simulink model "signal2Arduino"  (R2017a)
settings: Solver=ode3  StartTime=0.0  StopTime=T_end  FixedStep=Ts_sim  RelTol=1e-3  EnableMultiTasking=on
undefined symbols (not defined in the file or in its folder): A_butter_acc, A_butter_cal, A_butter_low, AD622, B_butter_acc, B_butter_cal, B_butter_low, b_stop, delta_EMG_RT, delta_theta1, EMG2vel_gain, g, Humusoft, input_type, k_stop, Ki_vel, Kp_vel, L_com, m1, m3, m_arm, min_EMG_RT, National_Instruments, PCI, phase_experiment, q1, q3, tau_max_cont, thetaL1_max, thetaL1_min, thetaR1_max, thetaR1_min, Ts_acc, Ts_sim, X, Y, Z
libraries: sm_lib x56, nesl_utility x23, sldrtlib x18, instrumentlib x2, simulink x1
(part 1 of 2)
settings Model: ExtModeTrigDuration=2  Creator=Fred Parietti  LastModifiedBy=jacob
settings DataIOCC: LimitDataPoints=on  SaveFormat=Array
settings OptimizationCC: LifeSpan=1
settings DebuggingCC: UnderspecifiedInitializationDetection=Classic  MergeDetectMultiDrivingBlocksExec=none  SFUnexpectedBacktrackingDiag=warning  SFNoUnconditionalDefaultTransitionDiag=warning  SFExecutionAtInitializationDiag=none
settings HardwareCC: ProdBitPerInt=16  ProdBitPerPointer=8  ProdBitPerSizeT=16  ProdBitPerPtrDiffT=16  ProdLargestAtomicFloat=None  ProdWordSize=8  ProdHWDeviceType=Atmel->AVR
settings ModelReferenceCC: PropagateSignalLabelsOutOfModel=off
settings SFSimCC: MATLABDynamicMemAlloc=off
settings RTWCC: SystemTargetFile=realtime.tlc  GenerateMakefile=off  TemplateMakefile=realtime.tmf  Description=Run on Target Hardware  RTWVerbose=off
settings STFCustomTargetCC: TargetLibSuffix=.a  GenerateSampleERTMain=on  ERTCustomFileBanners=on  SupportNonInlinedSFcns=off  RemoveResetFunc=on  SupportVariableSizeSignals=on  MATLABClassNameForMDSCustomization=Simulink.SoftwareTarget.ERTCustomization  GRTInterface=off  SystemTargetFile=realtime.tlc
settings ERTTargetCC: MultiwordLength=2048  GenerateSampleERTMain=on  ParMdlRefBuildCompliant=off  CompOptLevelCompliant=off  ConcurrentExecutionCompliant=off  CombineOutputUpdateFcns=off  ERTFirstTimeCompliant=off  SupportContinuousTime=on  SupportVariableSizeSignals=on  ModelStepFunctionPrototypeControlCompliant=off  CPPClassGenCompliant=off  UseToolchainInfoCompliant=off  ExtModeTransport=3  ExtModeMexFile=ext_serial_win32_comm_rtt  ExtModeMexArgs=0 1 9600  ERTSrcFileBannerTemplate=realtime_code_template.cgt  ERTHdrFileBannerTemplate=realtime_code_template.cgt  ERTDataSrcFileTemplate=realtime_code_template.cgt  ERTDataHdrFileTemplate=realtime_code_template.cgt  ERTCustomFileTemplate=realtime_file_process.tlc  ConvertIfToSwitch=off  SuppressUnreachableDefaultCases=off
settings ConfigComp: CovMetricSettings=dw  CovHtmlReporting=on  CovSaveCumulativeToWorkspaceVar=on  CovSaveSingleToWorkspaceVar=on  CovExternalEMLEnable=off
settings ConfigurationSet: Description=SimMechanics 2G
settings ExplorerConfigSet: InternalSimMechanicsExplorerSettings="<ExplorerConfiguration><canonicalview>planar_xy</canonicalview><AnimationSetting><BasePlaybackSpeed>1.0</BasePlaybackSpeed><PlaybackSpeedFactor>1.0</PlaybackSpeedFactor></AnimationSetting><TilePanel><TileInfo><Tiles Columns=\"1\" Count=\"1\" Rows=\"1\"><Column Left=\"2\" Weight=\"1\"/><Column Left=\"1036\"/><Row Top=\"2\" Weight=\"1\"/><Row Top=\"856\"/><Tile Height=\"1\" Width=\"1\" X=\"0\" Y=\"0\"/></Tiles></TileInfo><SceneInfo><SceneViewer><BGColor><R>1</R><G>1</G><B>1</B></BGColor><Camera><Position><X>1.1720425313593452</X><Y>1.5909414689803159</Y><Z>2.2841318134829445</Z></Position><Center><X>-0.16046430282016899</X><Y>0.25843463480080253</Y><Z>0.95162497930343193</Z></Center><Up><X>-0.40824829046386307</X><Y>0.81649658092772615</Y><Z>-0.40824829046386307</Z></Up><Left>-1.5455518852644918</Left><Right>1.5455518852644918</Right><Bottom>-1.165175562863084</Bottom><Top>1.165175562863084</Top></Camera></SceneViewer></SceneInfo></TilePanel></ExplorerConfiguration>"

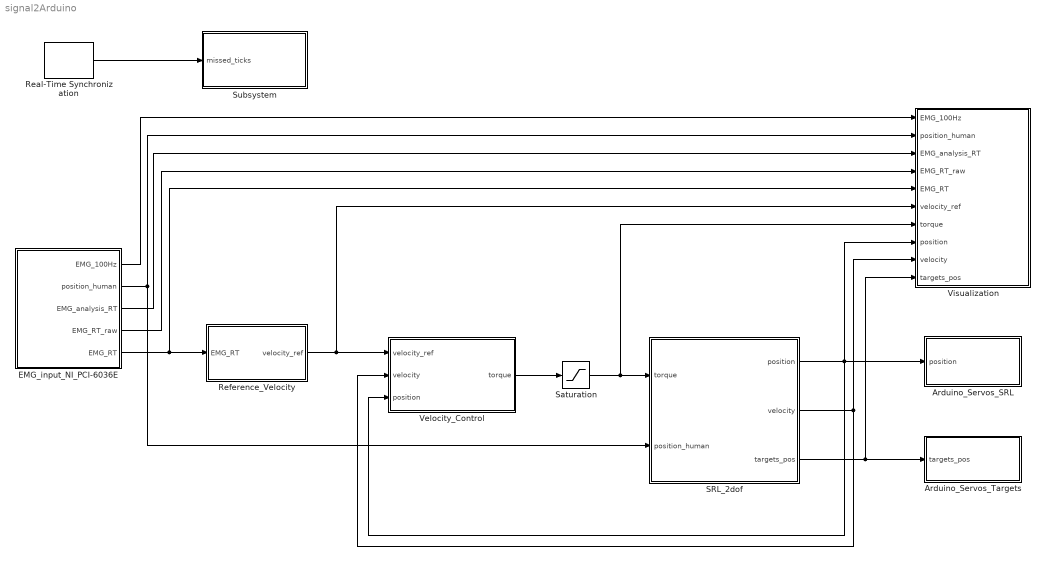
== system signal2Arduino ==
  Arduino_Servos_SRL : Subsystem
  Arduino_Servos_Targets : Subsystem
  EMG_input_NI_PCI-6036E : Subsystem
  Real-Time Synchronization : sldrtlib/Real-Time Synchronization  SampleTime=Ts_sim  MaxMissedTicks=10000  ShowMissedTicks=on  YieldWhenWaiting=off
  Reference_Velocity : Subsystem
  SRL_2dof : Subsystem
  Saturation : Saturate  UpperLimit=tau_max_cont  LowerLimit=-tau_max_cont
  Subsystem : Subsystem
  Velocity_Control : Subsystem
  Visualization : Subsystem
  wires:
  SRL_2dof/1(position) -> Velocity_Control/3(position), Arduino_Servos_SRL/1(position), Visualization/8(position)
  Saturation/1 -> Visualization/7(torque), SRL_2dof/1(torque)
  SRL_2dof/2(velocity) -> Velocity_Control/2(velocity), Visualization/9(velocity)
  Reference_Velocity/1(velocity_ref) -> Velocity_Control/1(velocity_ref), Visualization/6(velocity_ref)
  Velocity_Control/1(torque) -> Saturation/1
  EMG_input_NI_PCI-6036E/5(EMG_RT) -> Visualization/5(EMG_RT), Reference_Velocity/1(EMG_RT)
  Real-Time Synchronization/1 -> Subsystem/1(missed_ticks)
  SRL_2dof/3(targets_pos) -> Visualization/10(targets_pos), Arduino_Servos_Targets/1(targets_pos)
  EMG_input_NI_PCI-6036E/3(EMG_analysis_RT) -> Visualization/3(EMG_analysis_RT)
  EMG_input_NI_PCI-6036E/2(position_human) -> Visualization/2(position_human), SRL_2dof/2(position_human)
  EMG_input_NI_PCI-6036E/4(EMG_RT_raw) -> Visualization/4(EMG_RT_raw)
  EMG_input_NI_PCI-6036E/1(EMG_100Hz) -> Visualization/1(EMG_100Hz)

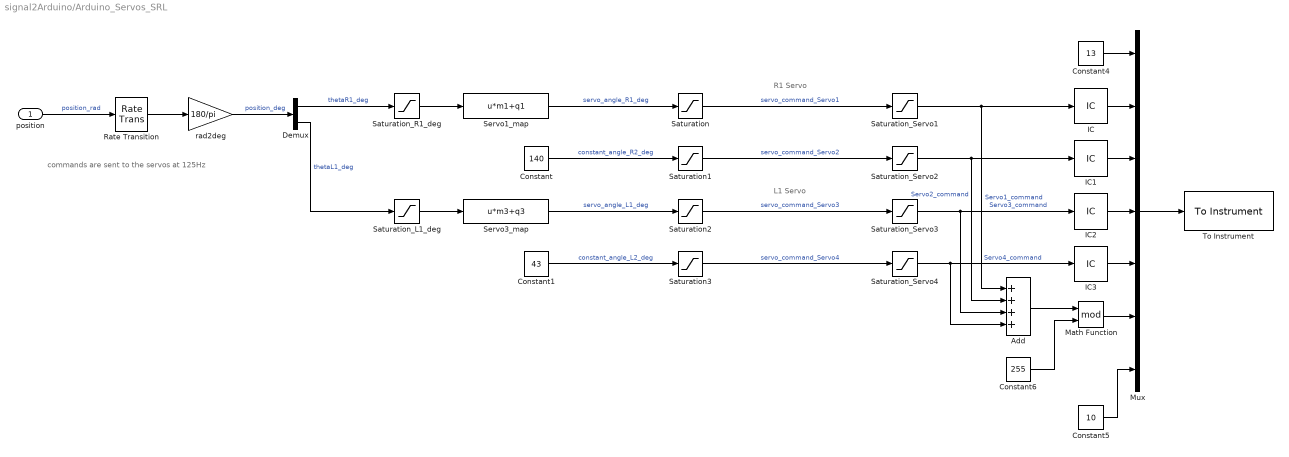
== system signal2Arduino/Arduino_Servos_SRL ==
  note: R1 Servo
  note: L1 Servo
  note: commands are sent to the servos at 125Hz
  position : Inport
  Add : Sum  Inputs=++++
  Constant : Constant  Value=140
  Constant1 : Constant  Value=43
  Constant4 : Constant  Value=13
  Constant5 : Constant  Value=10
  Constant6 : Constant  Value=255
  Demux : Demux  Outputs=2
  IC{,1..3} (4 alike) : InitialCondition  Value=90
  Math Function : Math  Operator=mod  SaturateOnIntegerOverflow=on
  Mux : Mux  Inputs=7
  Rate Transition : RateTransition  Deterministic=off  OutPortSampleTime=0.008
  Saturation : Saturate  UpperLimit=150  LowerLimit=23
  Saturation1 : Saturate  UpperLimit=140  LowerLimit=90
  Saturation2 : Saturate  UpperLimit=158  LowerLimit=30
  Saturation3 : Saturate  UpperLimit=93  LowerLimit=43
  Saturation_L1_deg : Saturate  UpperLimit=thetaL1_max/pi*180  LowerLimit=thetaL1_min/pi*180
  Saturation_R1_deg : Saturate  UpperLimit=thetaR1_max/pi*180  LowerLimit=thetaR1_min/pi*180
  Saturation_Servo{1..4} (4 alike) : Saturate  UpperLimit=180  LowerLimit=0
  Servo1_map : Fcn  Expr=u*m1+q1
  Servo3_map : Fcn  Expr=u*m3+q3
  To Instrument : instrumentlib/To Instrument  sampleTime=0.008  isWorkspaceObject=on  timeout=10  inputBufferSize=8192  protocol=Serial  serialPort=COM1  baudRate=9600  gpibVendor=Agilent Technologies  boardIndex=0  primaryAddress=1  secondaryAddress=0  visaVendor=Agilent  visaSerialPort=0  chassisIndex=0  logicalAddress=0  tcpRemoteHost='127.0.0.1'  tcpRemotePort=4500  udpRemoteHost='127.0.0.1'  udpRemotePort=9090  visaTCPBoardIndex=0  visaTCPRemoteHost='127.0.0.1'  usbBoardIndex=0  usbManufID=0  usbModelCode=0  usbSerialNumber=0  wsVariableName=s_SRL  initAction=None  initCommand='DATA:SOURCE CH1'  initFunction=get  command=''  sendFormat=Binary  asciiFormatting='%d'  precision=8-bit unsigned integer  byteOrder=Little endian
      settings: SourceProductName=Instrument Control Toolbox  SourceProductBaseCode=IC
  rad2deg : Gain  Gain=180/pi
  wires:
  position/1 -> Rate Transition/1  "position_rad"
  rad2deg/1 -> Demux/1  "position_deg"
  Demux/1 -> Saturation_R1_deg/1  "thetaR1_deg"
  Servo1_map/1 -> Saturation/1  "servo_angle_R1_deg"
  Demux/2 -> Saturation_L1_deg/1  "thetaL1_deg"
  Servo3_map/1 -> Saturation2/1  "servo_angle_L1_deg"
  Rate Transition/1 -> rad2deg/1
  Saturation/1 -> Saturation_Servo1/1  "servo_command_Servo1"
  Saturation1/1 -> Saturation_Servo2/1  "servo_command_Servo2"
  Saturation2/1 -> Saturation_Servo3/1  "servo_command_Servo3"
  Saturation3/1 -> Saturation_Servo4/1  "servo_command_Servo4"
  Constant/1 -> Saturation1/1  "constant_angle_R2_deg"
  Constant1/1 -> Saturation3/1  "constant_angle_L2_deg"
  Saturation_R1_deg/1 -> Servo1_map/1
  Saturation_L1_deg/1 -> Servo3_map/1
  Saturation_Servo4/1 -> IC3/1, Add/4  "Servo4_command"
  Saturation_Servo3/1 -> IC2/1, Add/3  "Servo3_command"
  Saturation_Servo2/1 -> IC1/1, Add/2  "Servo2_command"
  Saturation_Servo1/1 -> Add/1, IC/1  "Servo1_command"
  Math Function/1 -> Mux/6
  Constant4/1 -> Mux/1
  Constant6/1 -> Math Function/2
  Add/1 -> Math Function/1
  Constant5/1 -> Mux/7
  Mux/1 -> To Instrument/1
  IC/1 -> Mux/2
  IC1/1 -> Mux/3
  IC2/1 -> Mux/4
  IC3/1 -> Mux/5

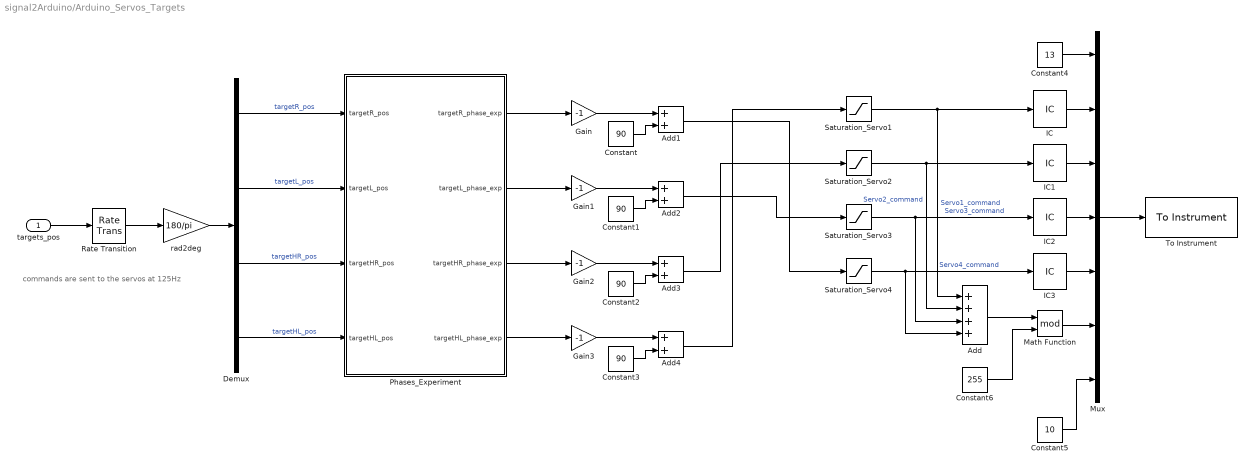
== system signal2Arduino/Arduino_Servos_Targets ==
  note: commands are sent to the servos at 125Hz
  targets_pos : Inport
  Add : Sum  Inputs=++++
  Add{1..4} (4 alike) : Sum
  Constant{,1..3} (4 alike) : Constant  Value=90
  Constant4 : Constant  Value=13
  Constant5 : Constant  Value=10
  Constant6 : Constant  Value=255
  Demux : Demux
  Gain{,1..3} (4 alike) : Gain  Gain=-1
  IC{,1..3} (4 alike) : InitialCondition  Value=90
  Math Function : Math  Operator=mod  SaturateOnIntegerOverflow=on
  Mux : Mux  Inputs=7
  Phases_Experiment : Subsystem
  Rate Transition : RateTransition  Deterministic=off  OutPortSampleTime=0.008
  Saturation_Servo{1..4} (4 alike) : Saturate  UpperLimit=180  LowerLimit=0
  To Instrument : instrumentlib/To Instrument  sampleTime=0.008  isWorkspaceObject=on  timeout=10  inputBufferSize=8192  protocol=Serial  serialPort=COM1  baudRate=9600  gpibVendor=Agilent Technologies  boardIndex=0  primaryAddress=1  secondaryAddress=0  visaVendor=Agilent  visaSerialPort=0  chassisIndex=0  logicalAddress=0  tcpRemoteHost='127.0.0.1'  tcpRemotePort=4500  udpRemoteHost='127.0.0.1'  udpRemotePort=9090  visaTCPBoardIndex=0  visaTCPRemoteHost='127.0.0.1'  usbBoardIndex=0  usbManufID=0  usbModelCode=0  usbSerialNumber=0  wsVariableName=s_targets  initAction=None  initCommand='DATA:SOURCE CH1'  initFunction=get  command=''  sendFormat=Binary  asciiFormatting='%d'  precision=8-bit unsigned integer  byteOrder=Little endian
      settings: SourceProductName=Instrument Control Toolbox  SourceProductBaseCode=IC
  rad2deg : Gain  Gain=180/pi
  wires:
  Saturation_Servo4/1 -> IC3/1, Add/4  "Servo4_command"
  Saturation_Servo3/1 -> IC2/1, Add/3  "Servo3_command"
  Saturation_Servo2/1 -> IC1/1, Add/2  "Servo2_command"
  Saturation_Servo1/1 -> Add/1, IC/1  "Servo1_command"
  Math Function/1 -> Mux/6
  Constant4/1 -> Mux/1
  Constant6/1 -> Math Function/2
  Add/1 -> Math Function/1
  Constant5/1 -> Mux/7
  Mux/1 -> To Instrument/1
  targets_pos/1 -> Rate Transition/1
  Demux/1 -> Phases_Experiment/1(targetR_pos)  "targetR_pos"
  Gain/1 -> Add1/1
  rad2deg/1 -> Demux/1
  Constant/1 -> Add1/2
  Gain1/1 -> Add2/1
  Constant1/1 -> Add2/2
  Gain2/1 -> Add3/1
  Constant2/1 -> Add3/2
  Gain3/1 -> Add4/1
  Constant3/1 -> Add4/2
  Demux/3 -> Phases_Experiment/3(targetHR_pos)  "targetHR_pos"
  Demux/2 -> Phases_Experiment/2(targetL_pos)  "targetL_pos"
  Demux/4 -> Phases_Experiment/4(targetHL_pos)  "targetHL_pos"
  Rate Transition/1 -> rad2deg/1
  IC/1 -> Mux/2
  IC1/1 -> Mux/3
  IC2/1 -> Mux/4
  IC3/1 -> Mux/5
  Add1/1 -> Saturation_Servo4/1
  Add2/1 -> Saturation_Servo3/1
  Add3/1 -> Saturation_Servo2/1
  Add4/1 -> Saturation_Servo1/1
  Phases_Experiment/1(targetR_phase_exp) -> Gain/1
  Phases_Experiment/2(targetL_phase_exp) -> Gain1/1
  Phases_Experiment/3(targetHR_phase_exp) -> Gain2/1
  Phases_Experiment/4(targetHL_phase_exp) -> Gain3/1

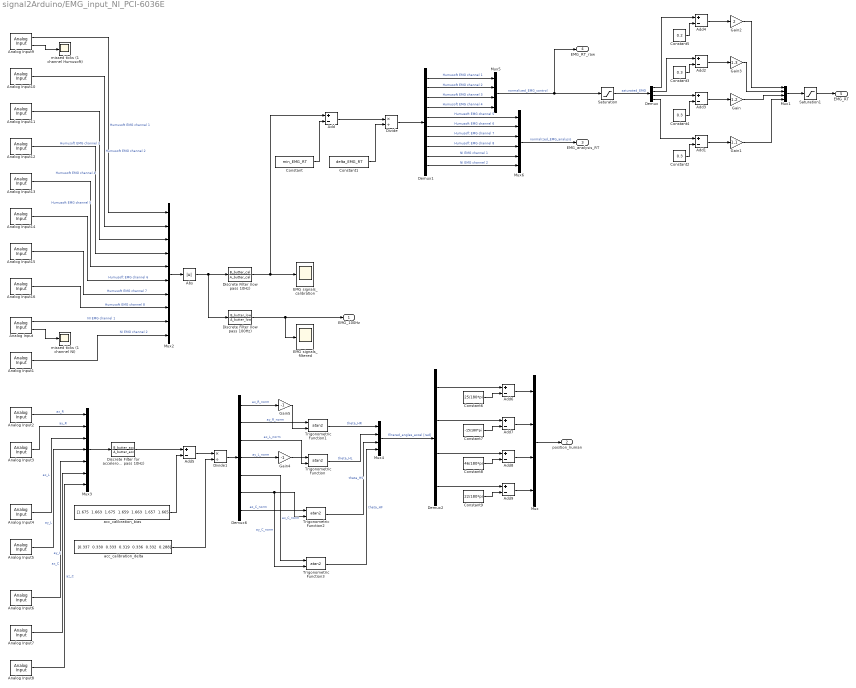
== system signal2Arduino/EMG_input_NI_PCI-6036E ==
  Abs : Abs
  Add{,1..9} (10 alike) : Sum  Inputs=+-
  Analog Input : sldrtlib/Analog Input  SampleTime=Ts_sim  MaxMissedTicks=10000  ShowMissedTicks=on  YieldWhenWaiting=off  DrvName=National_Instruments/PCI-6036E  DrvAddress=4294967295  DrvOptions=[0 0 0 0 0 0]  Channels=1  RangeMode=1  VoltRange=1  DataType=1
      settings: AttributesFormatString=National Instruments\nPCI-6036E [auto]  SourceProductName=Simulink Desktop Real-Time
  Analog Input1 : sldrtlib/Analog Input  SampleTime=Ts_sim  MaxMissedTicks=10000  ShowMissedTicks=off  YieldWhenWaiting=off  DrvName=National_Instruments/PCI-6036E  DrvAddress=4294967295  DrvOptions=[0 0 0 0 0 0]  Channels=2  RangeMode=1  VoltRange=1  DataType=1
      settings: AttributesFormatString=National Instruments\nPCI-6036E [auto]  SourceProductName=Simulink Desktop Real-Time
  Analog Input10 : sldrtlib/Analog Input  SampleTime=Ts_sim  MaxMissedTicks=10000  ShowMissedTicks=off  YieldWhenWaiting=off  DrvName=Humusoft/AD622  DrvAddress=4294967295  DrvOptions=zeros(1,0)  Channels=2  RangeMode=1  VoltRange=1  DataType=1
      settings: AttributesFormatString=Humusoft\nAD622 [auto]  SourceProductName=Simulink Desktop Real-Time
  Analog Input11 : sldrtlib/Analog Input  SampleTime=Ts_sim  MaxMissedTicks=10000  ShowMissedTicks=off  YieldWhenWaiting=off  DrvName=Humusoft/AD622  DrvAddress=4294967295  DrvOptions=zeros(1,0)  Channels=3  RangeMode=1  VoltRange=1  DataType=1
      settings: AttributesFormatString=Humusoft\nAD622 [auto]  SourceProductName=Simulink Desktop Real-Time
  Analog Input12 : sldrtlib/Analog Input  SampleTime=Ts_sim  MaxMissedTicks=10000  ShowMissedTicks=off  YieldWhenWaiting=off  DrvName=Humusoft/AD622  DrvAddress=4294967295  DrvOptions=zeros(1,0)  Channels=4  RangeMode=1  VoltRange=1  DataType=1
      settings: AttributesFormatString=Humusoft\nAD622 [auto]  SourceProductName=Simulink Desktop Real-Time
  Analog Input13 : sldrtlib/Analog Input  SampleTime=Ts_sim  MaxMissedTicks=10000  ShowMissedTicks=off  YieldWhenWaiting=off  DrvName=Humusoft/AD622  DrvAddress=4294967295  DrvOptions=zeros(1,0)  Channels=5  RangeMode=1  VoltRange=1  DataType=1
      settings: AttributesFormatString=Humusoft\nAD622 [auto]  SourceProductName=Simulink Desktop Real-Time
  Analog Input14 : sldrtlib/Analog Input  SampleTime=Ts_sim  MaxMissedTicks=10000  ShowMissedTicks=off  YieldWhenWaiting=off  DrvName=Humusoft/AD622  DrvAddress=4294967295  DrvOptions=zeros(1,0)  Channels=6  RangeMode=1  VoltRange=1  DataType=1
      settings: AttributesFormatString=Humusoft\nAD622 [auto]  SourceProductName=Simulink Desktop Real-Time
  Analog Input15 : sldrtlib/Analog Input  SampleTime=Ts_sim  MaxMissedTicks=10000  ShowMissedTicks=off  YieldWhenWaiting=off  DrvName=Humusoft/AD622  DrvAddress=4294967295  DrvOptions=zeros(1,0)  Channels=7  RangeMode=1  VoltRange=1  DataType=1
      settings: AttributesFormatString=Humusoft\nAD622 [auto]  SourceProductName=Simulink Desktop Real-Time
  Analog Input16 : sldrtlib/Analog Input  SampleTime=Ts_sim  MaxMissedTicks=10000  ShowMissedTicks=off  YieldWhenWaiting=off  DrvName=Humusoft/AD622  DrvAddress=4294967295  DrvOptions=zeros(1,0)  Channels=8  RangeMode=1  VoltRange=1  DataType=1
      settings: AttributesFormatString=Humusoft\nAD622 [auto]  SourceProductName=Simulink Desktop Real-Time
  Analog Input2 : sldrtlib/Analog Input  SampleTime=Ts_acc  MaxMissedTicks=10000  ShowMissedTicks=off  YieldWhenWaiting=off  DrvName=National_Instruments/PCI-6036E  DrvAddress=4294967295  DrvOptions=[0 0 0 0 0 0]  Channels=3  RangeMode=1  VoltRange=1  DataType=1
      settings: AttributesFormatString=National Instruments\nPCI-6036E [auto]  SourceProductName=Simulink Desktop Real-Time
  Analog Input3 : sldrtlib/Analog Input  SampleTime=Ts_acc  MaxMissedTicks=10000  ShowMissedTicks=off  YieldWhenWaiting=off  DrvName=National_Instruments/PCI-6036E  DrvAddress=4294967295  DrvOptions=[0 0 0 0 0 0]  Channels=4  RangeMode=1  VoltRange=1  DataType=1
      settings: AttributesFormatString=National Instruments\nPCI-6036E [auto]  SourceProductName=Simulink Desktop Real-Time
  Analog Input4 : sldrtlib/Analog Input  SampleTime=Ts_acc  MaxMissedTicks=10000  ShowMissedTicks=off  YieldWhenWaiting=off  DrvName=National_Instruments/PCI-6036E  DrvAddress=4294967295  DrvOptions=[0 0 0 0 0 0]  Channels=5  RangeMode=1  VoltRange=1  DataType=1
      settings: AttributesFormatString=National Instruments\nPCI-6036E [auto]  SourceProductName=Simulink Desktop Real-Time
  Analog Input5 : sldrtlib/Analog Input  SampleTime=Ts_acc  MaxMissedTicks=10000  ShowMissedTicks=off  YieldWhenWaiting=off  DrvName=National_Instruments/PCI-6036E  DrvAddress=4294967295  DrvOptions=[0 0 0 0 0 0]  Channels=6  RangeMode=1  VoltRange=1  DataType=1
      settings: AttributesFormatString=National Instruments\nPCI-6036E [auto]  SourceProductName=Simulink Desktop Real-Time
  Analog Input6 : sldrtlib/Analog Input  SampleTime=Ts_acc  MaxMissedTicks=10000  ShowMissedTicks=off  YieldWhenWaiting=off  DrvName=National_Instruments/PCI-6036E  DrvAddress=4294967295  DrvOptions=[0 0 0 0 0 0]  Channels=7  RangeMode=1  VoltRange=1  DataType=1
      settings: AttributesFormatString=National Instruments\nPCI-6036E [auto]  SourceProductName=Simulink Desktop Real-Time
  Analog Input7 : sldrtlib/Analog Input  SampleTime=Ts_acc  MaxMissedTicks=10000  ShowMissedTicks=off  YieldWhenWaiting=off  DrvName=National_Instruments/PCI-6036E  DrvAddress=4294967295  DrvOptions=[0 0 0 0 0 0]  Channels=8  RangeMode=1  VoltRange=1  DataType=1
      settings: AttributesFormatString=National Instruments\nPCI-6036E [auto]  SourceProductName=Simulink Desktop Real-Time
  Analog Input8 : sldrtlib/Analog Input  SampleTime=Ts_acc  MaxMissedTicks=10000  ShowMissedTicks=off  YieldWhenWaiting=off  DrvName=National_Instruments/PCI-6036E  DrvAddress=4294967295  DrvOptions=[0 0 0 0 0 0]  Channels=16  RangeMode=1  VoltRange=1  DataType=1
      settings: AttributesFormatString=National Instruments\nPCI-6036E [auto]  SourceProductName=Simulink Desktop Real-Time
  Analog Input9 : sldrtlib/Analog Input  SampleTime=Ts_sim  MaxMissedTicks=10000  ShowMissedTicks=on  YieldWhenWaiting=off  DrvName=Humusoft/AD622  DrvAddress=4294967295  DrvOptions=zeros(1,0)  Channels=1  RangeMode=1  VoltRange=1  DataType=1
      settings: AttributesFormatString=Humusoft\nAD622 [auto]  SourceProductName=Simulink Desktop Real-Time
  Constant : Constant  Value=min_EMG_RT
  Constant1 : Constant  Value=delta_EMG_RT
  Constant2 : Constant  Value=0.3
  Constant3 : Constant  Value=0.3
  Constant4 : Constant  Value=0.3
  Constant5 : Constant  Value=0.2
  Constant6 : Constant  Value=25/180*pi
  Constant7 : Constant  Value=-15/180*pi
  Constant8 : Constant  Value=46/180*pi
  Constant9 : Constant  Value=22/180*pi
  Demux : Demux
  Demux1 : Demux  Outputs=10
  Demux2 : Demux
  Demux6 : Demux  Outputs=7
  Discrete Filter (low pass 100Hz) : DiscreteFilter  Numerator=B_butter_low  Denominator=A_butter_low
  Discrete Filter (low pass 10Hz) : DiscreteFilter  Numerator=B_butter_cal  Denominator=A_butter_cal
  Discrete Filter for accelerometers (low pass 10Hz) : DiscreteFilter  Numerator=B_butter_acc  Denominator=A_butter_acc
  Divide : Product  Inputs=*/
  Divide1 : Product  Inputs=*/
  EMG signals_calibration : Scope
  EMG signals_filtered : Scope
  Gain : Gain  Gain=1.2
  Gain1 : Gain  Gain=1.1
  Gain2 : Gain  Gain=2
  Gain3 : Gain  Gain=1.3
  Gain4 : Gain  Gain=-1
  Gain5 : Gain  Gain=-1
  Mux{,1,4..5} (4 alike) : Mux
  Mux2 : Mux  Inputs=10
  Mux3 : Mux  Inputs=7
  Mux6 : Mux  Inputs=6
  Saturation : Saturate  UpperLimit=1  LowerLimit=0
  Saturation1 : Saturate  UpperLimit=1  LowerLimit=0
  Trigonometric Function{,1..3} (4 alike) : Trigonometry  Operator=atan2
  acc_calibration_bias : Constant  Value="[1.675  1.663  1.675  1.659  1.663  1.657  1.665]"
  acc_calibration_delta : Constant  Value="[0.337  0.330  0.333  0.319  0.336  0.332  0.288]"
  missed ticks (1 channel Humusoft) : Scope
  missed ticks (1 channel NI) : Scope
  EMG_100Hz : Outport
  position_human : Outport  Port=2
  EMG_analysis_RT : Outport  Port=3
  EMG_RT_raw : Outport  Port=4
  EMG_RT : Outport  Port=5
  wires:
  Constant/1 -> Add/2
  Add/1 -> Divide/1
  Constant1/1 -> Divide/2
  Saturation/1 -> Demux/1  "saturated_EMG"
  Demux/4 -> Add1/1
  Constant2/1 -> Add1/2
  Demux/1 -> Add4/1
  Add1/1 -> Gain1/1
  Mux1/1 -> Saturation1/1
  Demux/2 -> Add2/1
  Constant3/1 -> Add2/2
  Add2/1 -> Gain3/1
  Saturation1/1 -> EMG_RT/1
  Demux/3 -> Add3/1
  Add3/1 -> Gain/1
  Constant4/1 -> Add3/2
  Constant5/1 -> Add4/2
  Add4/1 -> Gain2/1
  Gain/1 -> Mux1/3
  Gain1/1 -> Mux1/4
  Gain2/1 -> Mux1/1
  Gain3/1 -> Mux1/2
  Analog Input/1 -> Mux2/9  "NI EMG channel 1"
  Analog Input/2 -> missed ticks (1 channel NI)/1
  Analog Input1/1 -> Mux2/10  "NI EMG channel 2"
  Discrete Filter (low pass 10Hz)/1 -> Add/1, EMG signals_calibration/1
  Mux3/1 -> Discrete Filter for accelerometers (low pass 10Hz)/1
  Demux6/3 -> Trigonometric Function/2  "ax_L_norm"
  Demux6/4 -> Gain4/1  "ay_L_norm"
  Gain4/1 -> Trigonometric Function/1
  Trigonometric Function/1 -> Mux4/2  "theta_HL"
  Add5/1 -> Divide1/1
  Demux6/1 -> Gain5/1  "ax_R_norm"
  Demux6/2 -> Trigonometric Function1/1  "ay_R_norm"
  Trigonometric Function1/1 -> Mux4/1  "theta_HR"
  Divide1/1 -> Demux6/1
  Gain5/1 -> Trigonometric Function1/2
  Demux6/5 -> Trigonometric Function3/1  "ax_C_norm"
  Demux6/6 -> Trigonometric Function3/2, Trigonometric Function2/2  "ay_C_norm"
  Demux6/7 -> Trigonometric Function2/1  "az_C_norm"
  Trigonometric Function2/1 -> Mux4/3  "theta_HS"
  Trigonometric Function3/1 -> Mux4/4  "theta_HF"
  Analog Input2/1 -> Mux3/1  "ax_R"
  Analog Input3/1 -> Mux3/2  "ay_R"
  Analog Input4/1 -> Mux3/3  "ax_L"
  Analog Input5/1 -> Mux3/4  "ay_L"
  Analog Input6/1 -> Mux3/5  "ax_C"
  Analog Input7/1 -> Mux3/6  "ay_C"
  Analog Input8/1 -> Mux3/7  "az_C"
  Mux2/1 -> Abs/1
  Analog Input9/2 -> missed ticks (1 channel Humusoft)/1
  Analog Input9/1 -> Mux2/1  "Humusoft EMG channel 1"
  Analog Input10/1 -> Mux2/2  "Humusoft EMG channel 2"
  Analog Input11/1 -> Mux2/3  "Humusoft EMG channel 3"
  Analog Input12/1 -> Mux2/4  "Humusoft EMG channel 4"
  Analog Input13/1 -> Mux2/5  "Humusoft EMG channel 5"
  Analog Input16/1 -> Mux2/8  "Humusoft EMG channel 8"
  Analog Input14/1 -> Mux2/6  "Humusoft EMG channel 6"
  Analog Input15/1 -> Mux2/7  "Humusoft EMG channel 7"
  Mux4/1 -> Demux2/1  "filtered_angles_accel [rad]"
  Discrete Filter for accelerometers (low pass 10Hz)/1 -> Add5/1
  Abs/1 -> Discrete Filter (low pass 10Hz)/1, Discrete Filter (low pass 100Hz)/1
  Discrete Filter (low pass 100Hz)/1 -> EMG_100Hz/1, EMG signals_filtered/1
  Demux1/1 -> Mux5/1  "Humusoft EMG channel 1"
  Demux1/2 -> Mux5/2  "Humusoft EMG channel 2"
  Demux1/3 -> Mux5/3  "Humusoft EMG channel 3"
  Demux1/4 -> Mux5/4  "Humusoft EMG channel 4"
  Mux5/1 -> EMG_RT_raw/1, Saturation/1  "normalized_EMG_control"
  Demux1/5 -> Mux6/1  "Humusoft EMG channel 5"
  Demux1/10 -> Mux6/6  "NI EMG channel 2"
  Demux1/6 -> Mux6/2  "Humusoft EMG channel 6"
  Demux1/7 -> Mux6/3  "Humusoft EMG channel 7"
  Demux1/8 -> Mux6/4  "Humusoft EMG channel 8"
  Demux1/9 -> Mux6/5  "NI EMG channel 1"
  Mux6/1 -> EMG_analysis_RT/1  "normalized_EMG_analysis"
  Divide/1 -> Demux1/1
  acc_calibration_bias/1 -> Add5/2
  acc_calibration_delta/1 -> Divide1/2
  Mux/1 -> position_human/1
  Demux2/1 -> Add6/1
  Constant6/1 -> Add6/2
  Demux2/2 -> Add7/1
  Constant7/1 -> Add7/2
  Constant8/1 -> Add8/2
  Constant9/1 -> Add9/2
  Demux2/3 -> Add8/1
  Demux2/4 -> Add9/1
  Add6/1 -> Mux/1
  Add9/1 -> Mux/4
  Add7/1 -> Mux/2
  Add8/1 -> Mux/3

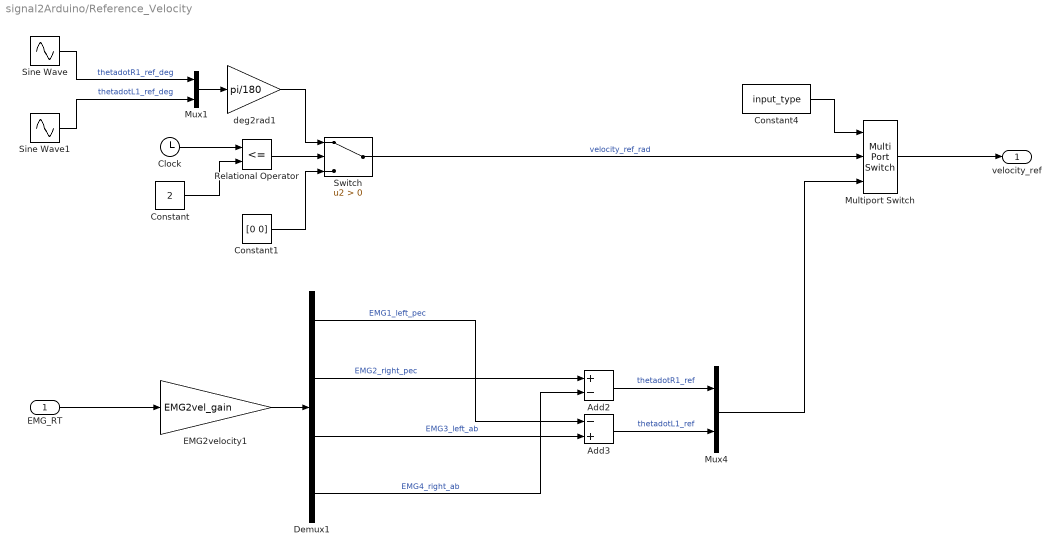
== system signal2Arduino/Reference_Velocity ==
  EMG_RT : Inport
  Add2 : Sum  Inputs=+-
  Add3 : Sum  Inputs=-+
  Clock : Clock
  Constant : Constant  Value=2
  Constant1 : Constant  Value=[0 0]
  Constant4 : Constant  Value=input_type
  Demux1 : Demux
  EMG2velocity1 : Gain  Gain=EMG2vel_gain
  Multiport Switch : MultiPortSwitch  Inputs=2
  Mux1 : Mux  Inputs=2
  Mux4 : Mux  Inputs=2
  Relational Operator : RelationalOperator  Operator=<=  OutDataTypeStr=boolean  RndMeth=Nearest
  Sine Wave : Sin  Amplitude=-40  Frequency=2*pi/(4)  SampleTime=0
  Sine Wave1 : Sin  Amplitude=-40  Frequency=2*pi/(4)  SampleTime=0
  Switch : Switch  Criteria=u2 > Threshold
  deg2rad1 : Gain  Gain=pi/180
  velocity_ref : Outport
  wires:
  Sine Wave/1 -> Mux1/1  "thetadotR1_ref_deg"
  Mux1/1 -> deg2rad1/1
  Switch/1 -> Multiport Switch/2  "velocity_ref_rad"
  Clock/1 -> Relational Operator/1
  Constant1/1 -> Switch/3
  Constant/1 -> Relational Operator/2
  Relational Operator/1 -> Switch/2
  deg2rad1/1 -> Switch/1
  Sine Wave1/1 -> Mux1/2  "thetadotL1_ref_deg"
  Constant4/1 -> Multiport Switch/1
  Multiport Switch/1 -> velocity_ref/1
  EMG2velocity1/1 -> Demux1/1
  Demux1/1 -> Add3/1  "EMG1_left_pec"
  Demux1/2 -> Add2/1  "EMG2_right_pec"
  Demux1/3 -> Add3/2  "EMG3_left_ab"
  Demux1/4 -> Add2/2  "EMG4_right_ab"
  Add2/1 -> Mux4/1  "thetadotR1_ref"
  Add3/1 -> Mux4/2  "thetadotL1_ref"
  EMG_RT/1 -> EMG2velocity1/1
  Mux4/1 -> Multiport Switch/3

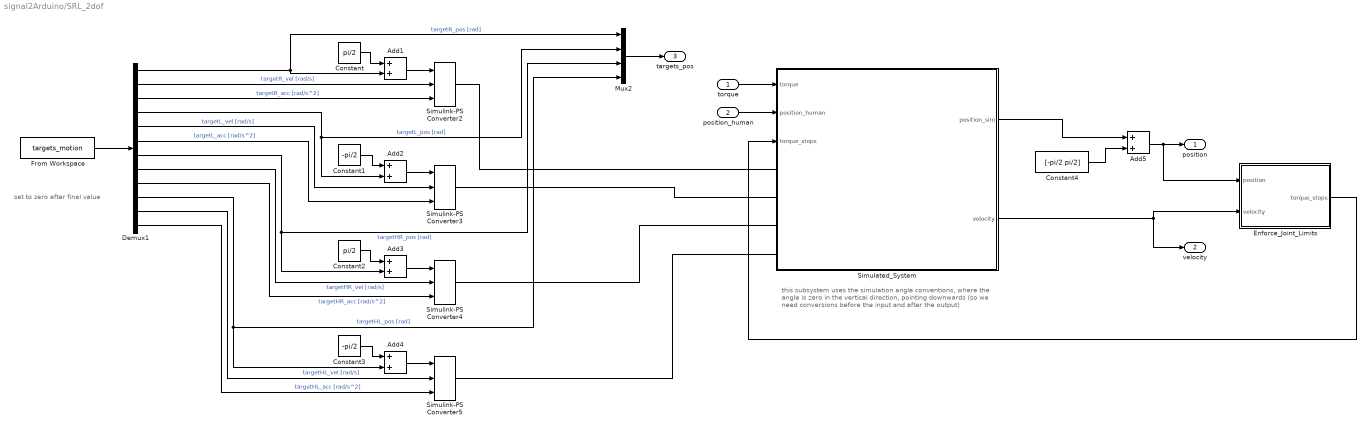
== system signal2Arduino/SRL_2dof ==
  note: this subsystem uses the simulation angle conventions, where the
      | angle is zero in the vertical direction, pointing downwards
      | (so we need conversions before the input and after the output)
  note: set to zero after final value
  torque : Inport
  position_human : Inport  Port=2
  Add{1..5} (5 alike) : Sum
  Constant : Constant  Value=pi/2
  Constant1 : Constant  Value=-pi/2
  Constant2 : Constant  Value=pi/2
  Constant3 : Constant  Value=-pi/2
  Constant4 : Constant  Value=[-pi/2 pi/2]
  Demux1 : Demux  Outputs=12
  Enforce_Joint_Limits : Subsystem
  From Workspace : FromWorkspace  VariableName=targets_motion  SampleTime=0  OutputAfterFinalValue=Setting to zero
  Mux2 : Mux
  Simulated_System : Subsystem
  Simulink-PS Converter{2..5} (4 alike) : nesl_utility/Simulink-PS Converter  PhysicalDomain=network_engine_domain  SubClassName=ps_input  LeftPortType=input  RightPortType=output  PseudoPeriodic=off  Frequencies=[]  NoiseDistribution=none  NoiseParameters=[]  Unit=1  AffineConversion=off  FilteringAndDerivatives=provide  SimscapeFilterOrder=1  InputFilterTimeConstant=0.001  UdotUserProvided=2
  position : Outport
  velocity : Outport  Port=2
  targets_pos : Outport  Port=3
  wires:
  From Workspace/1 -> Demux1/1
  Demux1/2 -> Simulink-PS Converter2/2  "targetR_vel [rad/s]"
  Demux1/3 -> Simulink-PS Converter2/3  "targetR_acc [rad/s^2]"
  Demux1/4 -> Add2/2, Mux2/2  "targetL_pos [rad]"
  Demux1/5 -> Simulink-PS Converter3/2  "targetL_vel [rad/s]"
  Demux1/6 -> Simulink-PS Converter3/3  "targetL_acc [rad/s^2]"
  Mux2/1 -> targets_pos/1
  Demux1/7 -> Mux2/3, Add3/2  "targetHR_pos [rad]"
  Demux1/8 -> Simulink-PS Converter4/2  "targetHR_vel [rad/s]"
  Demux1/9 -> Simulink-PS Converter4/3  "targetHR_acc [rad/s^2]"
  Demux1/10 -> Mux2/4, Add4/2  "targetHL_pos [rad]"
  Demux1/11 -> Simulink-PS Converter5/2  "targetHL_vel [rad/s]"
  Demux1/12 -> Simulink-PS Converter5/3  "targetHL_acc [rad/s^2]"
  Add1/1 -> Simulink-PS Converter2/1
  Constant/1 -> Add1/1
  Demux1/1 -> Add1/2, Mux2/1  "targetR_pos [rad]"
  Add2/1 -> Simulink-PS Converter3/1
  Constant1/1 -> Add2/1
  Constant2/1 -> Add3/1
  Add3/1 -> Simulink-PS Converter4/1
  Constant3/1 -> Add4/1
  Add4/1 -> Simulink-PS Converter5/1
  Constant4/1 -> Add5/2
  Simulated_System/2(velocity) -> Enforce_Joint_Limits/2(velocity), velocity/1
  torque/1 -> Simulated_System/1(torque)
  Enforce_Joint_Limits/1(torque_stops) -> Simulated_System/3(torque_stops)
  Simulated_System/1(position_sim) -> Add5/1
  Add5/1 -> Enforce_Joint_Limits/1(position), position/1
  position_human/1 -> Simulated_System/2(position_human)
  connections:
  Simulink-PS Converter2/RConn1 -- Simulated_System/LConn1
  Simulink-PS Converter3/RConn1 -- Simulated_System/LConn2
  Simulink-PS Converter4/RConn1 -- Simulated_System/LConn3
  Simulink-PS Converter5/RConn1 -- Simulated_System/LConn4

== system signal2Arduino/Subsystem ==
  missed_ticks : Inport
  Clock : Clock
  Compare To Constant : simulink/Logic and Bit Operations/Compare To Constant  relop=>  const=1  OutDataTypeStr=boolean
  Data Type Conversion : DataTypeConversion  OutDataTypeStr=double
  Gain : Gain  Gain=1/Ts_sim
  Integrator : Integrator  ExternalReset=rising
  missed ticks (total) : Scope
  sum of missed ticks : Scope
  wires:
  Gain/1 -> sum of missed ticks/1
  Compare To Constant/1 -> Integrator/2
  missed_ticks/1 -> Data Type Conversion/1, missed ticks (total)/1
  Data Type Conversion/1 -> Integrator/1
  Clock/1 -> Compare To Constant/1
  Integrator/1 -> Gain/1

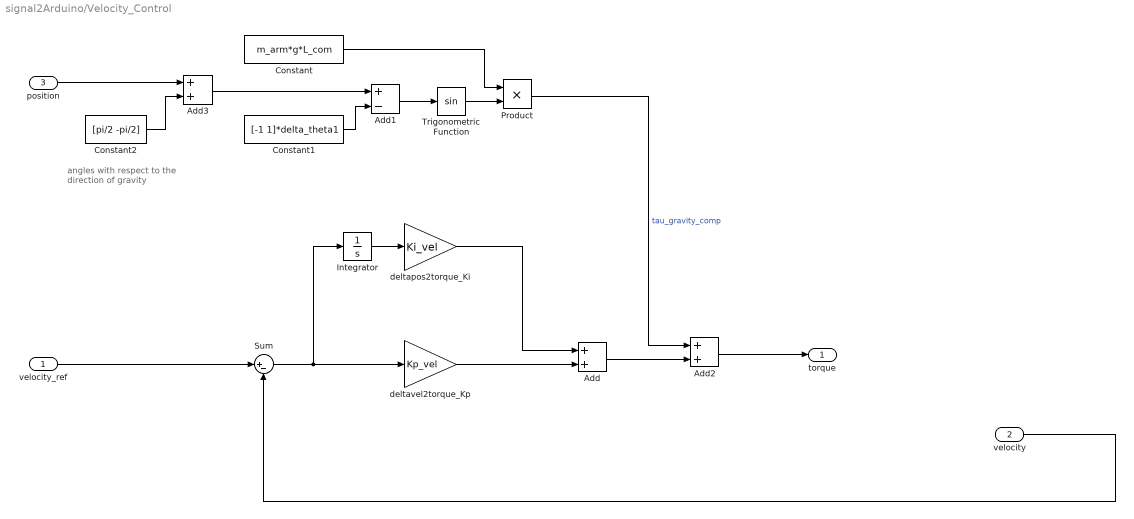
== system signal2Arduino/Velocity_Control ==
  note: angles with respect to
      | the direction of gravity
  velocity_ref : Inport
  velocity : Inport  Port=2
  position : Inport  Port=3
  Add : Sum
  Add1 : Sum  Inputs=+-
  Add2 : Sum
  Add3 : Sum
  Constant : Constant  Value=m_arm*g*L_com
  Constant1 : Constant  Value=[-1 1]*delta_theta1
  Constant2 : Constant  Value=[pi/2 -pi/2]
  Integrator : Integrator
  Product : Product
  Sum : Sum  Inputs=|+-
  Trigonometric Function : Trigonometry
  deltapos2torque_Ki : Gain  Gain=Ki_vel
  deltavel2torque_Kp : Gain  Gain=Kp_vel
  torque : Outport
  wires:
  velocity_ref/1 -> Sum/1
  velocity/1 -> Sum/2
  Sum/1 -> deltavel2torque_Kp/1, Integrator/1
  deltavel2torque_Kp/1 -> Add/2
  deltapos2torque_Ki/1 -> Add/1
  Add/1 -> Add2/2
  Integrator/1 -> deltapos2torque_Ki/1
  position/1 -> Add3/1
  Constant1/1 -> Add1/2
  Add1/1 -> Trigonometric Function/1
  Constant/1 -> Product/1
  Trigonometric Function/1 -> Product/2
  Product/1 -> Add2/1  "tau_gravity_comp"
  Add2/1 -> torque/1
  Add3/1 -> Add1/1
  Constant2/1 -> Add3/2

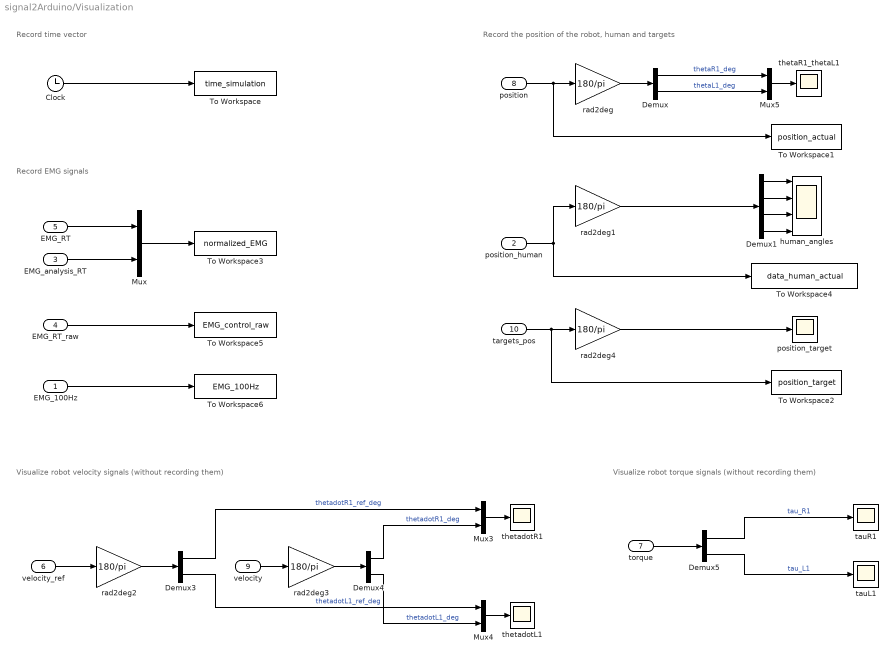
== system signal2Arduino/Visualization ==
  note: Record time vector
  note: Record EMG signals
  note: Record the position of the robot, human and targets
  note: Visualize robot velocity signals (without recording them)
  note: Visualize robot torque signals (without recording them)
  EMG_100Hz : Inport
  position_human : Inport  Port=2
  EMG_analysis_RT : Inport  Port=3
  EMG_RT_raw : Inport  Port=4
  EMG_RT : Inport  Port=5
  velocity_ref : Inport  Port=6
  torque : Inport  Port=7
  position : Inport  Port=8
  velocity : Inport  Port=9
  targets_pos : Inport  Port=10
  Clock : Clock
  Demux{,3..5} (4 alike) : Demux  Outputs=2
  Demux1 : Demux
  Mux{,3..5} (4 alike) : Mux  Inputs=2
  To Workspace : ToWorkspace  VariableName=time_simulation  SampleTime=-1
  To Workspace1 : ToWorkspace  VariableName=position_actual  SampleTime=-1
  To Workspace2 : ToWorkspace  VariableName=position_target  SampleTime=-1
  To Workspace3 : ToWorkspace  VariableName=normalized_EMG  SampleTime=-1
  To Workspace4 : ToWorkspace  VariableName=data_human_actual  SaveFormat=Structure With Time  SampleTime=-1
  To Workspace5 : ToWorkspace  VariableName=EMG_control_raw  SampleTime=-1
  To Workspace6 : ToWorkspace  VariableName=EMG_100Hz  SampleTime=-1
  human_angles : Scope  NumInputPorts=4
  position_target : Scope
  rad2deg{,1..4} (5 alike) : Gain  Gain=180/pi
  tauL1 : Scope
  tauR1 : Scope
  thetaR1_thetaL1 : Scope
  thetadotL1 : Scope
  thetadotR1 : Scope
  wires:
  Demux/2 -> Mux5/2  "thetaL1_deg"
  position/1 -> rad2deg/1, To Workspace1/1
  torque/1 -> Demux5/1
  Demux5/2 -> tauL1/1  "tau_L1"
  Demux5/1 -> tauR1/1  "tau_R1"
  rad2deg/1 -> Demux/1
  Demux/1 -> Mux5/1  "thetaR1_deg"
  velocity_ref/1 -> rad2deg2/1
  rad2deg2/1 -> Demux3/1
  velocity/1 -> rad2deg3/1
  Mux3/1 -> thetadotR1/1
  Demux3/1 -> Mux3/1  "thetadotR1_ref_deg"
  rad2deg3/1 -> Demux4/1
  Demux4/1 -> Mux3/2  "thetadotR1_deg"
  Mux4/1 -> thetadotL1/1
  Demux4/2 -> Mux4/2  "thetadotL1_deg"
  Demux3/2 -> Mux4/1  "thetadotL1_ref_deg"
  Clock/1 -> To Workspace/1
  Mux5/1 -> thetaR1_thetaL1/1
  EMG_RT/1 -> Mux/1
  targets_pos/1 -> To Workspace2/1, rad2deg4/1
  EMG_analysis_RT/1 -> Mux/2
  Mux/1 -> To Workspace3/1
  position_human/1 -> To Workspace4/1, rad2deg1/1
  rad2deg1/1 -> Demux1/1
  Demux1/4 -> human_angles/4
  Demux1/3 -> human_angles/3
  Demux1/2 -> human_angles/2
  Demux1/1 -> human_angles/1
  rad2deg4/1 -> position_target/1
  EMG_RT_raw/1 -> To Workspace5/1
  EMG_100Hz/1 -> To Workspace6/1

== system signal2Arduino/Arduino_Servos_Targets/Phases_Experiment ==
  targetR_pos : Inport
  targetL_pos : Inport  Port=2
  targetHR_pos : Inport  Port=3
  targetHL_pos : Inport  Port=4
  Constant : Constant  Value=-60
  Constant1 : Constant  Value=60
  Constant3 : Constant  Value=60
  Constant5 : Constant  Value=-60
  Constant7 : Constant  Value=phase_experiment
  Multiport Switch{,1..3} (4 alike) : MultiPortSwitch
  targetR_phase_exp : Outport
  targetL_phase_exp : Outport  Port=2
  targetHR_phase_exp : Outport  Port=3
  targetHL_phase_exp : Outport  Port=4
  wires:
  Constant7/1 -> Multiport Switch/1, Multiport Switch3/1, Multiport Switch2/1, Multiport Switch1/1
  Constant/1 -> Multiport Switch/2  "[deg]"
  targetR_pos/1 -> Multiport Switch/3, Multiport Switch/4  "[deg]"
  Multiport Switch/1 -> targetR_phase_exp/1
  Constant1/1 -> Multiport Switch1/2  "[deg]"
  targetL_pos/1 -> Multiport Switch1/4, Multiport Switch1/3  "[deg]"
  Multiport Switch1/1 -> targetL_phase_exp/1
  targetHR_pos/1 -> Multiport Switch2/2, Multiport Switch2/4  "[deg]"
  Multiport Switch2/1 -> targetHR_phase_exp/1
  Constant3/1 -> Multiport Switch2/3  "[deg]"
  targetHL_pos/1 -> Multiport Switch3/4, Multiport Switch3/2  "[deg]"
  Multiport Switch3/1 -> targetHL_phase_exp/1
  Constant5/1 -> Multiport Switch3/3  "[deg]"

== system signal2Arduino/SRL_2dof/Enforce_Joint_Limits ==
  position : Inport
  velocity : Inport  Port=2
  Constant : Constant  Value=thetaR1_max
  Constant1 : Constant  Value=thetaL1_max
  Constant2 : Constant  Value=thetaR1_min
  Constant3 : Constant  Value=thetaL1_min
  Demux : Demux  Outputs=2
  Demux1 : Demux  Outputs=2
  Joint_Limits : Subsystem
  Joint_Limits1 : Subsystem
  Mux : Mux  Inputs=2
  torque_stops : Outport
  wires:
  position/1 -> Demux/1
  velocity/1 -> Demux1/1
  Demux1/1 -> Joint_Limits/2(joint_velocity)  "thetadotR1_rad"
  Constant/1 -> Joint_Limits/3(limit_max)
  Demux/1 -> Joint_Limits/1(joint_position)  "thetaR1_rad"
  Constant2/1 -> Joint_Limits/4(limit_min)
  Joint_Limits/1(tau_stop) -> Mux/1  "tauR1_stop"
  Mux/1 -> torque_stops/1  "tau_stop"
  Demux1/2 -> Joint_Limits1/2(joint_velocity)  "thetadotL1_rad"
  Demux/2 -> Joint_Limits1/1(joint_position)  "thetaL1_rad"
  Constant1/1 -> Joint_Limits1/3(limit_max)
  Constant3/1 -> Joint_Limits1/4(limit_min)
  Joint_Limits1/1(tau_stop) -> Mux/2  "tauL1_stop"

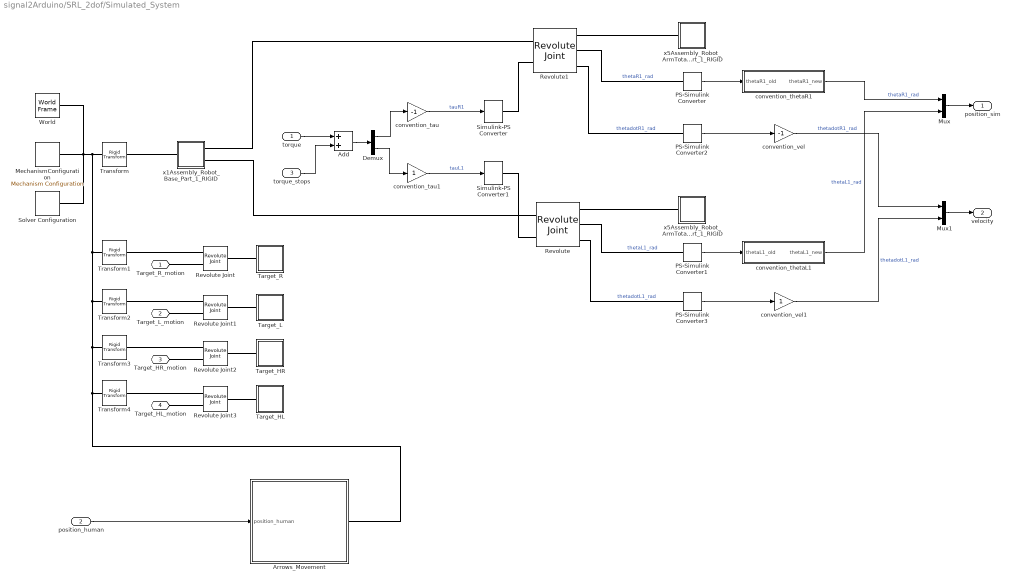
== system signal2Arduino/SRL_2dof/Simulated_System ==
  torque : Inport
  position_human : Inport  Port=2
  torque_stops : Inport  Port=3
  Add : Sum
  Arrows_Movement : Subsystem
  Demux : Demux  Outputs=2
  MechanismConfiguration : sm_lib/Utilities/Mechanism Configuration  UniformGravity=Constant  GravityVector=[0 -9.81 0]  GravityUnits=m/s^2  LinearizationDelta=0.001
  Mux : Mux  Inputs=2
  Mux1 : Mux  Inputs=2
  PS-Simulink Converter{,1..3} (4 alike) : nesl_utility/PS-Simulink Converter  PhysicalDomain=network_engine_domain  SubClassName=ps_output  LeftPortType=input  RightPortType=output  PseudoPeriodic=off  Frequencies=[]  Unit=1  AffineConversion=off
  Revolute : sm_lib/Joints/Revolute Joint  SenseConstraintForce=off  SenseConstraintForceX=off  SenseConstraintForceY=off  SenseConstraintForceZ=off  SenseConstraintTorque=off  SenseConstraintTorqueX=off  SenseConstraintTorqueY=off  SenseConstraintTorqueZ=off  SenseTotalForce=off  SenseTotalForceX=off  SenseTotalForceY=off  SenseTotalForceZ=off  SenseTotalTorque=off  SenseTotalTorqueX=off  SenseTotalTorqueY=off  SenseTotalTorqueZ=off  CompositeWrenchDir=FollowerOnBase  CompositeWrenchFrame=BaseFrame  EquilibriumPosition=0  EquilibriumPositionUnits=rad  SpringStiffness=0  SpringStiffnessUnits=m*N/rad  DampingCoefficient=0  DampingCoefficientUnits=m*s*N/rad  TorqueActuationMode=InputTorque  MotionActuationMode=ComputedMotion  SensePosition=on  SenseVelocity=on  SenseAcceleration=off  SenseTorqueForce=off  PositionTargetSpecify=on  PositionTargetPriority=Low  PositionTargetValue=0  PositionTargetValueUnits=deg  VelocityTargetSpecify=off  VelocityTargetPriority=High  VelocityTargetValue=0  VelocityTargetValueUnits=deg/s
  Revolute Joint : sm_lib/Joints/Revolute Joint  SenseConstraintForce=off  SenseConstraintForceX=off  SenseConstraintForceY=off  SenseConstraintForceZ=off  SenseConstraintTorque=off  SenseConstraintTorqueX=off  SenseConstraintTorqueY=off  SenseConstraintTorqueZ=off  SenseTotalForce=off  SenseTotalForceX=off  SenseTotalForceY=off  SenseTotalForceZ=off  SenseTotalTorque=off  SenseTotalTorqueX=off  SenseTotalTorqueY=off  SenseTotalTorqueZ=off  CompositeWrenchDir=FollowerOnBase  CompositeWrenchFrame=BaseFrame  EquilibriumPosition=0  EquilibriumPositionUnits=deg  SpringStiffness=0  SpringStiffnessUnits=N*m/deg  DampingCoefficient=0  DampingCoefficientUnits=N*m/(deg/s)  TorqueActuationMode=ComputedTorque  MotionActuationMode=InputMotion  SensePosition=off  SenseVelocity=off  SenseAcceleration=off  SenseTorqueForce=off  PositionTargetSpecify=on  PositionTargetPriority=Low  PositionTargetValue=90  PositionTargetValueUnits=deg  VelocityTargetSpecify=off  VelocityTargetPriority=High  VelocityTargetValue=0  VelocityTargetValueUnits=deg/s
  Revolute Joint1 : sm_lib/Joints/Revolute Joint  SenseConstraintForce=off  SenseConstraintForceX=off  SenseConstraintForceY=off  SenseConstraintForceZ=off  SenseConstraintTorque=off  SenseConstraintTorqueX=off  SenseConstraintTorqueY=off  SenseConstraintTorqueZ=off  SenseTotalForce=off  SenseTotalForceX=off  SenseTotalForceY=off  SenseTotalForceZ=off  SenseTotalTorque=off  SenseTotalTorqueX=off  SenseTotalTorqueY=off  SenseTotalTorqueZ=off  CompositeWrenchDir=FollowerOnBase  CompositeWrenchFrame=BaseFrame  EquilibriumPosition=0  EquilibriumPositionUnits=deg  SpringStiffness=0  SpringStiffnessUnits=N*m/deg  DampingCoefficient=0  DampingCoefficientUnits=N*m/(deg/s)  TorqueActuationMode=ComputedTorque  MotionActuationMode=InputMotion  SensePosition=off  SenseVelocity=off  SenseAcceleration=off  SenseTorqueForce=off  PositionTargetSpecify=on  PositionTargetPriority=Low  PositionTargetValue=-90  PositionTargetValueUnits=deg  VelocityTargetSpecify=off  VelocityTargetPriority=High  VelocityTargetValue=0  VelocityTargetValueUnits=deg/s
  Revolute Joint2 : sm_lib/Joints/Revolute Joint  SenseConstraintForce=off  SenseConstraintForceX=off  SenseConstraintForceY=off  SenseConstraintForceZ=off  SenseConstraintTorque=off  SenseConstraintTorqueX=off  SenseConstraintTorqueY=off  SenseConstraintTorqueZ=off  SenseTotalForce=off  SenseTotalForceX=off  SenseTotalForceY=off  SenseTotalForceZ=off  SenseTotalTorque=off  SenseTotalTorqueX=off  SenseTotalTorqueY=off  SenseTotalTorqueZ=off  CompositeWrenchDir=FollowerOnBase  CompositeWrenchFrame=BaseFrame  EquilibriumPosition=0  EquilibriumPositionUnits=deg  SpringStiffness=0  SpringStiffnessUnits=N*m/deg  DampingCoefficient=0  DampingCoefficientUnits=N*m/(deg/s)  TorqueActuationMode=ComputedTorque  MotionActuationMode=InputMotion  SensePosition=off  SenseVelocity=off  SenseAcceleration=off  SenseTorqueForce=off  PositionTargetSpecify=on  PositionTargetPriority=Low  PositionTargetValue=90  PositionTargetValueUnits=deg  VelocityTargetSpecify=off  VelocityTargetPriority=High  VelocityTargetValue=0  VelocityTargetValueUnits=deg/s
  Revolute Joint3 : sm_lib/Joints/Revolute Joint  SenseConstraintForce=off  SenseConstraintForceX=off  SenseConstraintForceY=off  SenseConstraintForceZ=off  SenseConstraintTorque=off  SenseConstraintTorqueX=off  SenseConstraintTorqueY=off  SenseConstraintTorqueZ=off  SenseTotalForce=off  SenseTotalForceX=off  SenseTotalForceY=off  SenseTotalForceZ=off  SenseTotalTorque=off  SenseTotalTorqueX=off  SenseTotalTorqueY=off  SenseTotalTorqueZ=off  CompositeWrenchDir=FollowerOnBase  CompositeWrenchFrame=BaseFrame  EquilibriumPosition=0  EquilibriumPositionUnits=deg  SpringStiffness=0  SpringStiffnessUnits=N*m/deg  DampingCoefficient=0  DampingCoefficientUnits=N*m/(deg/s)  TorqueActuationMode=ComputedTorque  MotionActuationMode=InputMotion  SensePosition=off  SenseVelocity=off  SenseAcceleration=off  SenseTorqueForce=off  PositionTargetSpecify=on  PositionTargetPriority=Low  PositionTargetValue=-90  PositionTargetValueUnits=deg  VelocityTargetSpecify=off  VelocityTargetPriority=High  VelocityTargetValue=0  VelocityTargetValueUnits=deg/s
  Revolute1 : sm_lib/Joints/Revolute Joint  SenseConstraintForce=off  SenseConstraintForceX=off  SenseConstraintForceY=off  SenseConstraintForceZ=off  SenseConstraintTorque=off  SenseConstraintTorqueX=off  SenseConstraintTorqueY=off  SenseConstraintTorqueZ=off  SenseTotalForce=off  SenseTotalForceX=off  SenseTotalForceY=off  SenseTotalForceZ=off  SenseTotalTorque=off  SenseTotalTorqueX=off  SenseTotalTorqueY=off  SenseTotalTorqueZ=off  CompositeWrenchDir=FollowerOnBase  CompositeWrenchFrame=BaseFrame  EquilibriumPosition=0  EquilibriumPositionUnits=rad  SpringStiffness=0  SpringStiffnessUnits=m*N/rad  DampingCoefficient=0  DampingCoefficientUnits=m*s*N/rad  TorqueActuationMode=InputTorque  MotionActuationMode=ComputedMotion  SensePosition=on  SenseVelocity=on  SenseAcceleration=off  SenseTorqueForce=off  PositionTargetSpecify=on  PositionTargetPriority=Low  PositionTargetValue=0  PositionTargetValueUnits=deg  VelocityTargetSpecify=off  VelocityTargetPriority=High  VelocityTargetValue=0  VelocityTargetValueUnits=deg/s
  Simulink-PS Converter : nesl_utility/Simulink-PS Converter  PhysicalDomain=network_engine_domain  SubClassName=ps_input  LeftPortType=input  RightPortType=output  PseudoPeriodic=off  Frequencies=[]  NoiseDistribution=none  NoiseParameters=[]  Unit=1  AffineConversion=off  FilteringAndDerivatives=zero  SimscapeFilterOrder=1  InputFilterTimeConstant=0.001  UdotUserProvided=1
  Simulink-PS Converter1 : nesl_utility/Simulink-PS Converter  PhysicalDomain=network_engine_domain  SubClassName=ps_input  LeftPortType=input  RightPortType=output  PseudoPeriodic=off  Frequencies=[]  NoiseDistribution=none  NoiseParameters=[]  Unit=1  AffineConversion=off  FilteringAndDerivatives=zero  SimscapeFilterOrder=1  InputFilterTimeConstant=0.001  UdotUserProvided=1
  Solver Configuration : nesl_utility/Solver Configuration  PhysicalDomain=network_engine_domain  SubClassName=solver  LeftPortType=input  RightPortType=generic  Accelerate=off  Tones=[]  Harmonics=[]  SimulateNoise=off  Profile=off  UseLocalSampling=off  EnableSwitchedLinearOptims=on  FrequencyDomain=off  UseCCode=off  RelTol=0.001  AbsTol=1e-06  MinStep=1e-09  ToWorkspace=off  RevertToSquareIcSolve=off  NumHomotopyIterations=100  PhasorMode=off  PhasorModeNumHarmonics=1  OverrideAbsTol=off  DoDC=off  ResidualTolerance=1e-09  UseLocalSolver=off  LocalSolverChoice=NE_BACKWARD_EULER_ADVANCER  LocalSolverSampleTime=0.001  DoFixedCost=off  MaxNonlinIter=3  MaxModeIter=2  LinearAlgebra=Sparse  DelaysMemoryBudget=1024  AutomaticFiltering=on  FilteringTimeConstant=0.001
  Target_HL : Subsystem
  Target_HR : Subsystem
  Target_L : Subsystem
  Target_R : Subsystem
  Transform : sm_lib/Frames and Transforms/Rigid Transform  TranslationMethod=Cartesian  TranslationStandardOffset=0  TranslationLengthUnit=mm  TranslationStandardAxis=+Z  TranslationCartesianOffset=[-131.68773658972694 0 0]  TranslationROffset=0  TranslationROffsetUnits=m  TranslationZOffset=0  TranslationZOffsetUnits=m  TranslationThetaOffset=0  TranslationThetaOffsetUnits=deg  RotationMethod=ArbitraryAxis  RotationAngleUnits=rad  RotationStandardAxis=+Z  RotationAngle=0  RotationArbitraryAxis=[0 0 0]  FollAlignAxisA=+X  BaseAlignAxisA=+Y  FollAlignAxisB=+Y  BaseAlignAxisB=+Z  RotationSequenceAxes=FollowerAxes  RotationSequence=XYX  RotationSequenceAngles=[0 0 0]  RotationSequenceAnglesUnits=deg  RotationMatrix=[1 0 0; 0 1 0; 0 0 1]
  Transform1 : sm_lib/Frames and Transforms/Rigid Transform  TranslationMethod=Cartesian  TranslationStandardOffset=0  TranslationLengthUnit=mm  TranslationStandardAxis=+Z  TranslationCartesianOffset=[(-131.68773658972694-161.81641196165057) 220.50618817795822 393.1157122563057]  TranslationROffset=0  TranslationROffsetUnits=m  TranslationZOffset=0  TranslationZOffsetUnits=m  TranslationThetaOffset=0  TranslationThetaOffsetUnits=deg  RotationMethod=ArbitraryAxis  RotationAngleUnits=rad  RotationStandardAxis=+Z  RotationAngle=-pi/2  RotationArbitraryAxis=[0 1 0]  FollAlignAxisA=+X  BaseAlignAxisA=+Y  FollAlignAxisB=+Y  BaseAlignAxisB=+Z  RotationSequenceAxes=FollowerAxes  RotationSequence=XYX  RotationSequenceAngles=[0 0 0]  RotationSequenceAnglesUnits=deg  RotationMatrix=[1 0 0; 0 1 0; 0 0 1]
  Transform2 : sm_lib/Frames and Transforms/Rigid Transform  TranslationMethod=Cartesian  TranslationStandardOffset=0  TranslationLengthUnit=mm  TranslationStandardAxis=+Z  TranslationCartesianOffset=[(-131.68773658972694+417.19188514110454+7.999999999999886) 220.50618817795822 393.1157122563057]  TranslationROffset=0  TranslationROffsetUnits=m  TranslationZOffset=0  TranslationZOffsetUnits=m  TranslationThetaOffset=0  TranslationThetaOffsetUnits=deg  RotationMethod=ArbitraryAxis  RotationAngleUnits=rad  RotationStandardAxis=+Z  RotationAngle=pi/2  RotationArbitraryAxis=[0 1 0]  FollAlignAxisA=+X  BaseAlignAxisA=+Y  FollAlignAxisB=+Y  BaseAlignAxisB=+Z  RotationSequenceAxes=FollowerAxes  RotationSequence=XYX  RotationSequenceAngles=[0 0 0]  RotationSequenceAnglesUnits=deg  RotationMatrix=[1 0 0; 0 1 0; 0 0 1]
  Transform3 : sm_lib/Frames and Transforms/Rigid Transform  TranslationMethod=Cartesian  TranslationStandardOffset=0  TranslationLengthUnit=mm  TranslationStandardAxis=+Z  TranslationCartesianOffset=[(-131.68773658972694-161.81641196165057+150) 220.50618817795822 393.1157122563057]  TranslationROffset=0  TranslationROffsetUnits=m  TranslationZOffset=0  TranslationZOffsetUnits=m  TranslationThetaOffset=0  TranslationThetaOffsetUnits=deg  RotationMethod=ArbitraryAxis  RotationAngleUnits=rad  RotationStandardAxis=+Z  RotationAngle=-pi/2  RotationArbitraryAxis=[0 1 0]  FollAlignAxisA=+X  BaseAlignAxisA=+Y  FollAlignAxisB=+Y  BaseAlignAxisB=+Z  RotationSequenceAxes=FollowerAxes  RotationSequence=XYX  RotationSequenceAngles=[0 0 0]  RotationSequenceAnglesUnits=deg  RotationMatrix=[1 0 0; 0 1 0; 0 0 1]
  Transform4 : sm_lib/Frames and Transforms/Rigid Transform  TranslationMethod=Cartesian  TranslationStandardOffset=0  TranslationLengthUnit=mm  TranslationStandardAxis=+Z  TranslationCartesianOffset=[(-131.68773658972694+417.19188514110454+7.999999999999886-150) 220.50618817795822 393.1157122563057]  TranslationROffset=0  TranslationROffsetUnits=m  TranslationZOffset=0  TranslationZOffsetUnits=m  TranslationThetaOffset=0  TranslationThetaOffsetUnits=deg  RotationMethod=ArbitraryAxis  RotationAngleUnits=rad  RotationStandardAxis=+Z  RotationAngle=pi/2  RotationArbitraryAxis=[0 1 0]  FollAlignAxisA=+X  BaseAlignAxisA=+Y  FollAlignAxisB=+Y  BaseAlignAxisB=+Z  RotationSequenceAxes=FollowerAxes  RotationSequence=XYX  RotationSequenceAngles=[0 0 0]  RotationSequenceAnglesUnits=deg  RotationMatrix=[1 0 0; 0 1 0; 0 0 1]
  World : sm_lib/Frames and Transforms/World Frame
  convention_tau : Gain  Gain=-1
  convention_tau1 : Gain
  convention_thetaL1 : Subsystem
  convention_thetaR1 : Subsystem
  convention_vel : Gain  Gain=-1
  convention_vel1 : Gain
  x1Assembly_Robot_Base_Part_1_RIGID : Subsystem
  x5Assembly_Robot_ArmTotalShoulder_L_Part_1_RIGID : Subsystem
  x5Assembly_Robot_ArmTotalShoulder_R_Part_1_RIGID : Subsystem
  Target_R_motion : PMIOPort  Port=1  Side=Left
  Target_L_motion : PMIOPort  Port=2  Side=Left
  Target_HR_motion : PMIOPort  Port=3  Side=Left
  Target_HL_motion : PMIOPort  Port=4  Side=Left
  position_sim : Outport
  velocity : Outport  Port=2
  wires:
  PS-Simulink Converter/1 -> convention_thetaR1/1(thetaR1_old)
  PS-Simulink Converter1/1 -> convention_thetaL1/1(thetaL1_old)
  Mux/1 -> position_sim/1
  torque/1 -> Add/1
  Demux/1 -> convention_tau/1
  Demux/2 -> convention_tau1/1
  Mux1/1 -> velocity/1
  PS-Simulink Converter2/1 -> convention_vel/1
  PS-Simulink Converter3/1 -> convention_vel1/1
  Add/1 -> Demux/1
  torque_stops/1 -> Add/2
  convention_thetaR1/1(thetaR1_new) -> Mux/1  "thetaR1_rad"
  convention_thetaL1/1(thetaL1_new) -> Mux/2  "thetaL1_rad"
  convention_vel/1 -> Mux1/1  "thetadotR1_rad"
  convention_vel1/1 -> Mux1/2  "thetadotL1_rad"
  convention_tau/1 -> Simulink-PS Converter/1  "tauR1"
  convention_tau1/1 -> Simulink-PS Converter1/1  "tauL1"
  position_human/1 -> Arrows_Movement/1(position_human)
  connections:
  PS-Simulink Converter/LConn1 -- Revolute1/RConn2  "thetaR1_rad"
  Revolute/RConn2 -- PS-Simulink Converter1/LConn1  "thetaL1_rad"
  Revolute/LConn1 -- x1Assembly_Robot_Base_Part_1_RIGID/RConn2
  Revolute/RConn1 -- x5Assembly_Robot_ArmTotalShoulder_L_Part_1_RIGID/LConn1
  Transform/RConn1 -- x1Assembly_Robot_Base_Part_1_RIGID/LConn1
  Revolute1/LConn1 -- x1Assembly_Robot_Base_Part_1_RIGID/RConn1
  Revolute1/RConn1 -- x5Assembly_Robot_ArmTotalShoulder_R_Part_1_RIGID/LConn1
  Simulink-PS Converter/RConn1 -- Revolute1/LConn2
  Revolute/LConn2 -- Simulink-PS Converter1/RConn1
  Revolute1/RConn3 -- PS-Simulink Converter2/LConn1  "thetadotR1_rad"
  Revolute/RConn3 -- PS-Simulink Converter3/LConn1  "thetadotL1_rad"
  Transform1/RConn1 -- Revolute Joint/LConn1
  Revolute Joint/RConn1 -- Target_R/LConn1
  Target_R_motion/RConn1 -- Revolute Joint/LConn2
  Revolute Joint1/LConn1 -- Transform2/RConn1
  Revolute Joint1/RConn1 -- Target_L/LConn1
  Target_L_motion/RConn1 -- Revolute Joint1/LConn2
  Revolute Joint2/RConn1 -- Target_HR/LConn1
  Transform3/RConn1 -- Revolute Joint2/LConn1
  Revolute Joint3/RConn1 -- Target_HL/LConn1
  Revolute Joint3/LConn1 -- Transform4/RConn1
  Target_HR_motion/RConn1 -- Revolute Joint2/LConn2
  Target_HL_motion/RConn1 -- Revolute Joint3/LConn2
  MechanismConfiguration/RConn1 -- Arrows_Movement/RConn1 -- Transform4/LConn1 -- Transform3/LConn1 -- Transform2/LConn1 -- Transform1/LConn1 -- Transform/LConn1 -- Solver Configuration/RConn1 -- World/RConn1
